simulink model "sil_top"  (R2025b)
settings: Solver=FixedStepDiscrete  StartTime=0.0  StopTime=sil_t_final_s  FixedStep=0.01  RelTol=1e-3
undefined symbols (not defined in the file): sil_dt_s, sil_initial_sensor_packet
settings Model: Creator=O.Agaphonov  LastModifiedBy=O.Agaphonov

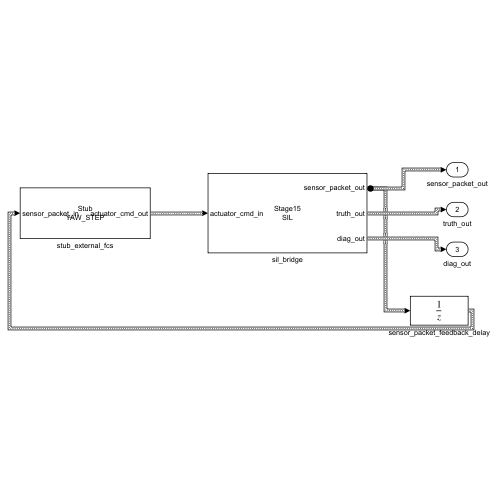
[thumbnail: Simulink's stored preview of the top-level diagram]
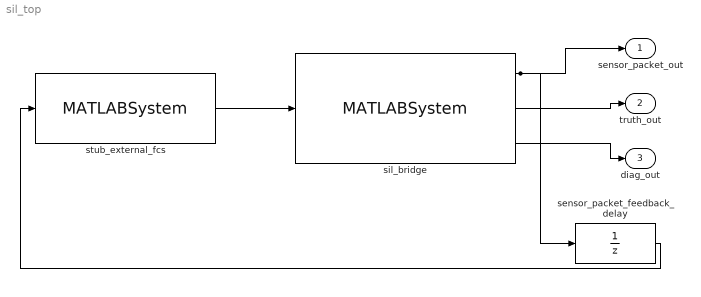
== system sil_top ==
  sensor_packet_feedback_delay : UnitDelay  InitialCondition=sil_initial_sensor_packet  SampleTime=sil_dt_s  HasFrameUpgradeWarning=on
  sil_bridge : MATLABSystem  System=uav.sl.Stage15SILBridgeSystem  dt_s=sil_dt_s  params=sil_params  state0=sil_state0  rates_cfg=sil_rates_cfg  time_s=sil_time_s  actuation_mode=norm01  SimulateUsing=Interpreted execution
      mask Type: uav.sl.Stage15SILBridgeSystem
  stub_external_fcs : MATLABSystem  System=uav.sl.StubExternalFCSSystem  mode_name=yaw_step  params=sil_params  SimulateUsing=Interpreted execution
      mask Type: uav.sl.StubExternalFCSSystem
  sensor_packet_out : Outport
  truth_out : Outport  Port=2
  diag_out : Outport  Port=3
  wires:
  stub_external_fcs/1 -> sil_bridge/1
  sil_bridge/1 -> sensor_packet_feedback_delay/1, sensor_packet_out/1
  sensor_packet_feedback_delay/1 -> stub_external_fcs/1
  sil_bridge/2 -> truth_out/1
  sil_bridge/3 -> diag_out/1
